simulink model "Midterm_Q4_sim"  (R2018b)
settings: Solver=VariableStepAuto  StartTime=0.0  StopTime=10.0  RelTol=1e-3
values from neighbouring files (symbols this model uses):
  A = [0 1;0 0]    [Midterm_Q4.m]
  C = [1 1]    [Midterm_Q4.m]
  K = [1;1]    [Midterm_Q4.m]
  x1filter = [1 0]    [Midterm_Q4.m]
settings Model: Creator=kiankhaneghahi  LastModifiedBy=kiankhaneghahi

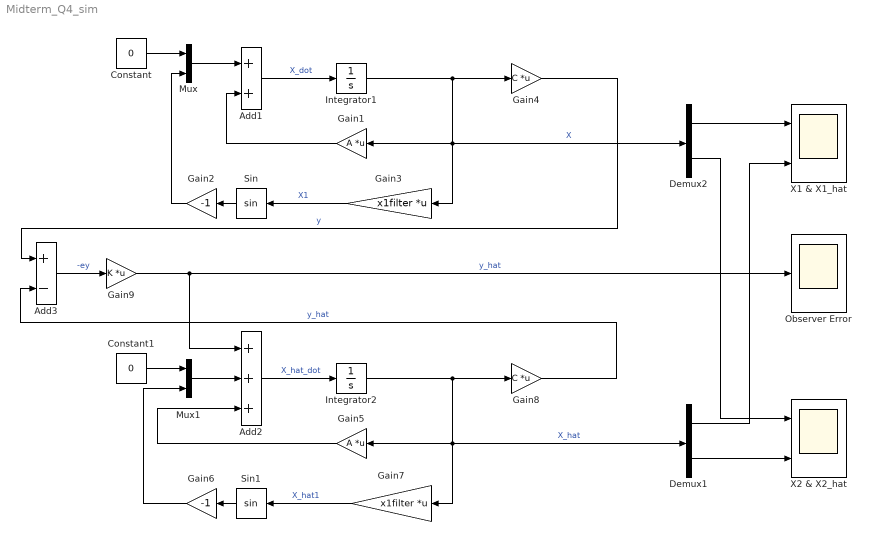
== system Midterm_Q4_sim ==
  Add1 : Sum
  Add2 : Sum  Inputs=+++
  Add3 : Sum  Inputs=+-
  Constant : Constant  Value=0
  Constant1 : Constant  Value=0
  Demux1 : Demux  Outputs=2
  Demux2 : Demux  Outputs=2
  Gain1 : Gain  Gain=A  Multiplication=Matrix(K*u)
  Gain2 : Gain  Gain=-1
  Gain3 : Gain  Gain=x1filter  Multiplication=Matrix(K*u)
  Gain4 : Gain  Gain=C  Multiplication=Matrix(K*u)
  Gain5 : Gain  Gain=A  Multiplication=Matrix(K*u)
  Gain6 : Gain  Gain=-1
  Gain7 : Gain  Gain=x1filter  Multiplication=Matrix(K*u)
  Gain8 : Gain  Gain=C  Multiplication=Matrix(K*u)
  Gain9 : Gain  Gain=K  Multiplication=Matrix(K*u)
  Integrator1 : Integrator  InitialCondition=[1 2]
  Integrator2 : Integrator  InitialCondition=[-1 3]
  Mux : Mux  Inputs=2
  Mux1 : Mux  Inputs=2
  Observer Error : Scope
  Sin : Trigonometry
  Sin1 : Trigonometry
  X1 & X1_hat : Scope  NumInputPorts=2
  X2 & X2_hat : Scope  NumInputPorts=2
  wires:
  Add1/1 -> Integrator1/1  "X_dot"
  Integrator1/1 -> Gain4/1, Demux2/1, Gain3/1, Gain1/1  "X"
  Gain1/1 -> Add1/2
  Gain3/1 -> Sin/1  "X1"
  Sin/1 -> Gain2/1
  Gain2/1 -> Mux/2
  Mux/1 -> Add1/1
  Constant/1 -> Mux/1
  Gain4/1 -> Add3/1  "y"
  Gain6/1 -> Mux1/2
  Gain8/1 -> Add3/2  "y_hat"
  Add2/1 -> Integrator2/1  "X_hat_dot"
  Constant1/1 -> Mux1/1
  Mux1/1 -> Add2/2
  Gain5/1 -> Add2/3
  Gain7/1 -> Sin1/1  "X_hat1"
  Sin1/1 -> Gain6/1
  Integrator2/1 -> Gain8/1, Demux1/1, Gain7/1, Gain5/1  "X_hat"
  Add3/1 -> Gain9/1  "-ey"
  Gain9/1 -> Observer Error/1, Add2/1  "y_hat"
  Demux2/1 -> X1 & X1_hat/1
  Demux1/1 -> X1 & X1_hat/2
  Demux2/2 -> X2 & X2_hat/1
  Demux1/2 -> X2 & X2_hat/2
